simulink model "stateflow_subchart_big"  (R2015b)
settings: Solver=VariableStepAuto  StartTime=0.0  StopTime=10.0  RelTol=1e-3
settings Model: Creator=ladmin  LastModifiedBy=ladmin

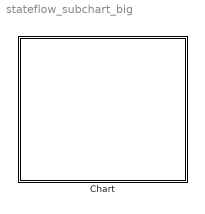
== system stateflow_subchart_big ==
  Chart : Stateflow chart  TreatAsAtomicUnit=on

== stateflow chart stateflow_subchart_big/Chart ==
  state Subchart
    state State_lvl2_2
    state State_lvl2_1
    State_lvl2_1 -> State_lvl2_2
  state State_lvl1
